simulink model "LAB_5"  (R2017b)
settings: Solver=VariableStepAuto  StartTime=0.0  StopTime=10  RelTol=1e-3
settings Model: Creator=maar  LastModifiedBy=maar

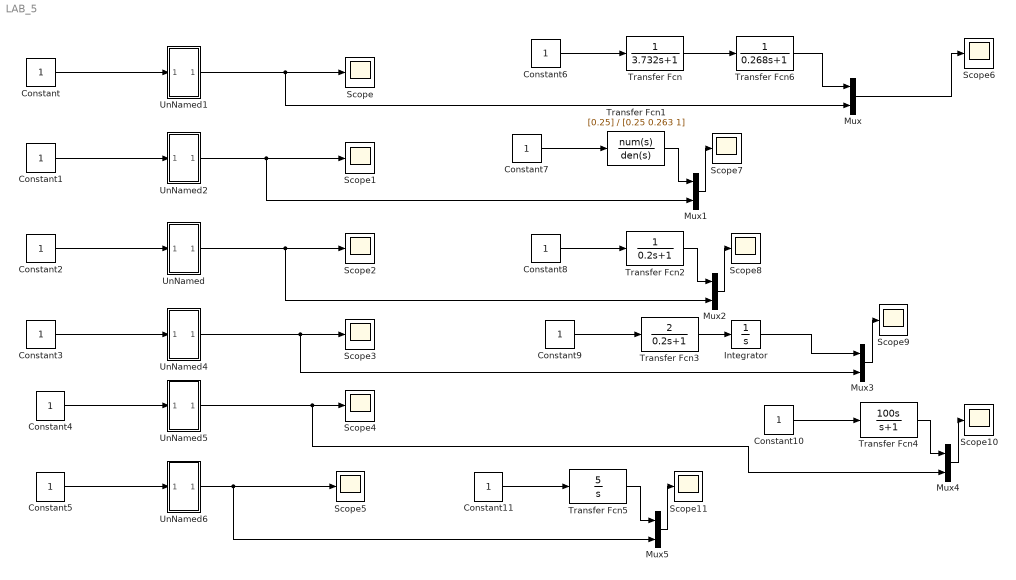
== system LAB_5 ==
  Constant{,1..11} (12 alike) : Constant
  Integrator : Integrator
  Mux{,1..5} (6 alike) : Mux  Inputs=2
  Scope{,1..11} (12 alike) : Scope
  Transfer Fcn : TransferFcn  Denominator=[3.732 1]
  Transfer Fcn1 : TransferFcn  Numerator=[0.25]  Denominator=[0.25 0.263 1]
  Transfer Fcn2 : TransferFcn  Denominator=[0.2 1]
  Transfer Fcn3 : TransferFcn  Numerator=[2]  Denominator=[0.2 1]
  Transfer Fcn4 : TransferFcn  Numerator=[100 0]  Denominator=[1 1]
  Transfer Fcn5 : TransferFcn  Numerator=[5]  Denominator=[1 0]
  Transfer Fcn6 : TransferFcn  Denominator=[0.268 1]
  UnNamed : Subsystem
  UnNamed1 : Subsystem
  UnNamed2 : Subsystem
  UnNamed4 : Subsystem
  UnNamed5 : Subsystem
  UnNamed6 : Subsystem
  wires:
  Constant/1 -> UnNamed1/1(in_1)
  Constant1/1 -> UnNamed2/1(in_1)
  Constant2/1 -> UnNamed/1(in_1)
  Constant3/1 -> UnNamed4/1(in_1)
  Constant4/1 -> UnNamed5/1(in_1)
  Constant5/1 -> UnNamed6/1(in_1)
  Constant6/1 -> Transfer Fcn/1
  UnNamed1/1(out_1) -> Mux/2, Scope/1
  Mux/1 -> Scope6/1
  UnNamed2/1(out_1) -> Mux1/2, Scope1/1
  Constant7/1 -> Transfer Fcn1/1
  Transfer Fcn1/1 -> Mux1/1
  Mux1/1 -> Scope7/1
  UnNamed/1(out_1) -> Mux2/2, Scope2/1
  Constant8/1 -> Transfer Fcn2/1
  Transfer Fcn2/1 -> Mux2/1
  Mux2/1 -> Scope8/1
  UnNamed4/1(out_1) -> Mux3/2, Scope3/1
  Constant9/1 -> Transfer Fcn3/1
  Mux3/1 -> Scope9/1
  UnNamed5/1(out_1) -> Mux4/2, Scope4/1
  Constant10/1 -> Transfer Fcn4/1
  Transfer Fcn4/1 -> Mux4/1
  Mux4/1 -> Scope10/1
  UnNamed6/1(out_1) -> Mux5/2, Scope5/1
  Constant11/1 -> Transfer Fcn5/1
  Transfer Fcn5/1 -> Mux5/1
  Mux5/1 -> Scope11/1
  Transfer Fcn/1 -> Transfer Fcn6/1
  Transfer Fcn6/1 -> Mux/1
  Transfer Fcn3/1 -> Integrator/1
  Integrator/1 -> Mux3/1

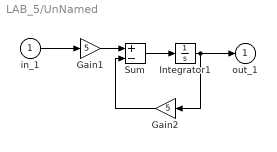
== system LAB_5/UnNamed ==
  in_1 : Inport
  Gain1 : Gain  Gain=5  SaturateOnIntegerOverflow=on  OutDataTypeStr=Inherit: Same as input  ParamDataTypeStr=Inherit: Same as input
  Gain2 : Gain  Gain=5  SaturateOnIntegerOverflow=on  OutDataTypeStr=Inherit: Same as input  ParamDataTypeStr=Inherit: Same as input
  Integrator1 : Integrator
  Sum : Sum  Inputs=+-  SaturateOnIntegerOverflow=on  InputSameDT=on  OutDataTypeStr=Inherit: Same as first input
  out_1 : Outport
  wires:
  in_1/1 -> Gain1/1
  Gain1/1 -> Sum/1
  Gain2/1 -> Sum/2
  Integrator1/1 -> Gain2/1, out_1/1
  Sum/1 -> Integrator1/1

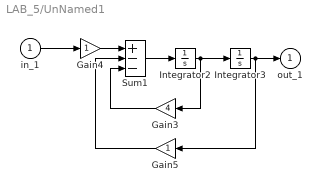
== system LAB_5/UnNamed1 ==
  in_1 : Inport
  Gain3 : Gain  Gain=4  SaturateOnIntegerOverflow=on  OutDataTypeStr=Inherit: Same as input  ParamDataTypeStr=Inherit: Same as input
  Gain4 : Gain  SaturateOnIntegerOverflow=on  OutDataTypeStr=Inherit: Same as input  ParamDataTypeStr=Inherit: Same as input
  Gain5 : Gain  SaturateOnIntegerOverflow=on  OutDataTypeStr=Inherit: Same as input  ParamDataTypeStr=Inherit: Same as input
  Integrator2 : Integrator
  Integrator3 : Integrator
  Sum1 : Sum  Inputs=+--  SaturateOnIntegerOverflow=on  InputSameDT=on  OutDataTypeStr=Inherit: Same as first input
  out_1 : Outport
  wires:
  Gain5/1 -> Sum1/2
  Integrator3/1 -> Gain5/1, out_1/1
  Integrator2/1 -> Integrator3/1, Gain3/1
  Gain3/1 -> Sum1/3
  in_1/1 -> Gain4/1
  Gain4/1 -> Sum1/1
  Sum1/1 -> Integrator2/1

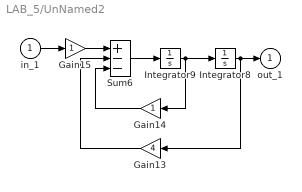
== system LAB_5/UnNamed2 ==
  in_1 : Inport
  Gain13 : Gain  Gain=4  SaturateOnIntegerOverflow=on  OutDataTypeStr=Inherit: Same as input  ParamDataTypeStr=Inherit: Same as input
  Gain14 : Gain  SaturateOnIntegerOverflow=on  OutDataTypeStr=Inherit: Same as input  ParamDataTypeStr=Inherit: Same as input
  Gain15 : Gain  SaturateOnIntegerOverflow=on  OutDataTypeStr=Inherit: Same as input  ParamDataTypeStr=Inherit: Same as input
  Integrator8 : Integrator
  Integrator9 : Integrator
  Sum6 : Sum  Inputs=+--  SaturateOnIntegerOverflow=on  InputSameDT=on  OutDataTypeStr=Inherit: Same as first input
  out_1 : Outport
  wires:
  Sum6/1 -> Integrator9/1
  Integrator9/1 -> Gain14/1, Integrator8/1
  Gain15/1 -> Sum6/1
  Gain14/1 -> Sum6/3
  Integrator8/1 -> out_1/1, Gain13/1
  Gain13/1 -> Sum6/2
  in_1/1 -> Gain15/1

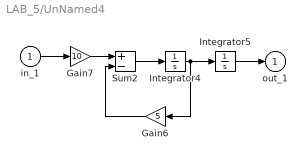
== system LAB_5/UnNamed4 ==
  in_1 : Inport
  Gain6 : Gain  Gain=5  SaturateOnIntegerOverflow=on  OutDataTypeStr=Inherit: Same as input  ParamDataTypeStr=Inherit: Same as input
  Gain7 : Gain  Gain=10  SaturateOnIntegerOverflow=on  OutDataTypeStr=Inherit: Same as input  ParamDataTypeStr=Inherit: Same as input
  Integrator4 : Integrator
  Integrator5 : Integrator
  Sum2 : Sum  Inputs=+-  SaturateOnIntegerOverflow=on  InputSameDT=on  OutDataTypeStr=Inherit: Same as first input
  out_1 : Outport
  wires:
  Gain7/1 -> Sum2/1
  Gain6/1 -> Sum2/2
  Integrator4/1 -> Gain6/1, Integrator5/1
  Sum2/1 -> Integrator4/1
  in_1/1 -> Gain7/1
  Integrator5/1 -> out_1/1

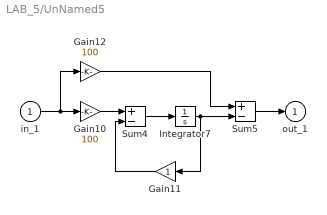
== system LAB_5/UnNamed5 ==
  in_1 : Inport
  Gain10 : Gain  Gain=100  SaturateOnIntegerOverflow=on  OutDataTypeStr=Inherit: Same as input  ParamDataTypeStr=Inherit: Same as input
  Gain11 : Gain  SaturateOnIntegerOverflow=on  OutDataTypeStr=Inherit: Same as input  ParamDataTypeStr=Inherit: Same as input
  Gain12 : Gain  Gain=100  SaturateOnIntegerOverflow=on  OutDataTypeStr=Inherit: Same as input  ParamDataTypeStr=Inherit: Same as input
  Integrator7 : Integrator
  Sum4 : Sum  Inputs=+-  SaturateOnIntegerOverflow=on  InputSameDT=on  OutDataTypeStr=Inherit: Same as first input
  Sum5 : Sum  Inputs=+-  SaturateOnIntegerOverflow=on  InputSameDT=on  OutDataTypeStr=Inherit: Same as first input
  out_1 : Outport
  wires:
  Gain12/1 -> Sum5/1
  in_1/1 -> Gain10/1, Gain12/1
  Gain10/1 -> Sum4/1
  Gain11/1 -> Sum4/2
  Integrator7/1 -> Gain11/1, Sum5/2
  Sum4/1 -> Integrator7/1
  Sum5/1 -> out_1/1

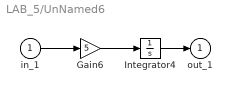
== system LAB_5/UnNamed6 ==
  in_1 : Inport
  Gain6 : Gain  Gain=5  SaturateOnIntegerOverflow=on  OutDataTypeStr=Inherit: Same as input  ParamDataTypeStr=Inherit: Same as input
  Integrator4 : Integrator
  out_1 : Outport
  wires:
  Gain6/1 -> Integrator4/1
  in_1/1 -> Gain6/1
  Integrator4/1 -> out_1/1
